simulink model "simulation_block"  (R2024b)
settings: Solver=VariableStepAuto  StartTime=0.0  StopTime=10.0  RelTol=1e-3
undefined symbols (not defined in the file or in its folder): r_min
settings Model: Creator=tianhaoji  LastModifiedBy=tianhaoji

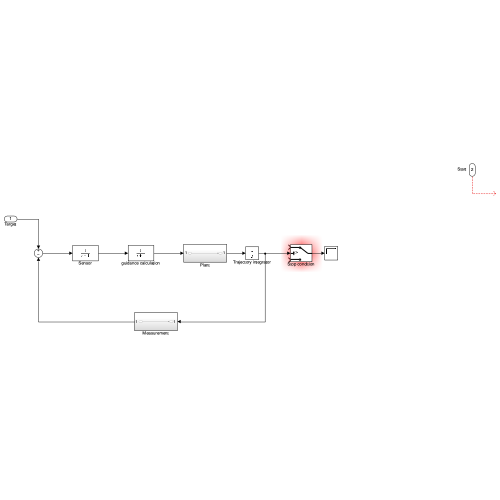
[thumbnail: Simulink's stored preview of the top-level diagram]
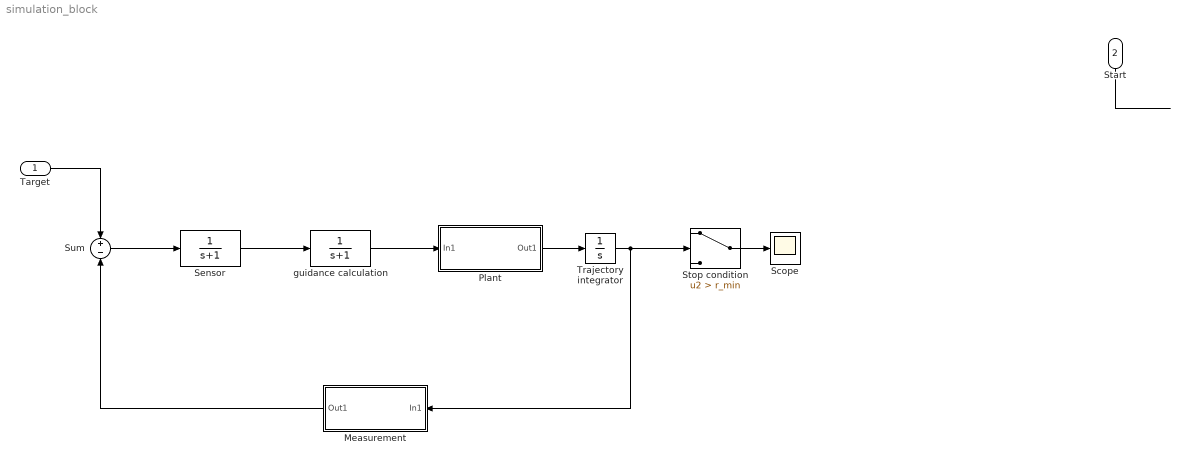
== system simulation_block ==
  Target : Inport
  Start : Inport  Port=2
  Measurement : Subsystem
  Plant : Subsystem
  Scope : Scope
  Sensor : TransferFcn  Denominator=[1 1]
  Stop condition : Switch  Criteria=u2 > Threshold  Threshold=r_min  SaturateOnIntegerOverflow=off  InputSameDT=off
  Sum : Sum  Inputs=+-
  Trajectory integrator : Integrator
  guidance calculation : TransferFcn  Denominator=[1 1]
  wires:
  Target/1 -> Sum/1
  Sum/1 -> Sensor/1
  Sensor/1 -> guidance calculation/1
  guidance calculation/1 -> Plant/1(In1)
  Plant/1(Out1) -> Trajectory integrator/1
  Trajectory integrator/1 -> Stop condition/2, Measurement/1(In1)
  Measurement/1(Out1) -> Sum/2
  Start/1 -> ?
  Stop condition/1 -> Scope/1

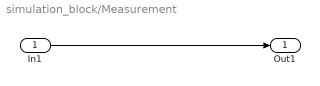
== system simulation_block/Measurement ==
  In1 : Inport
  Out1 : Outport
  wires:
  In1/1 -> Out1/1

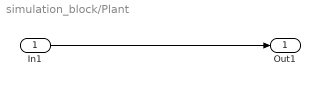
== system simulation_block/Plant ==
  In1 : Inport
  Out1 : Outport
  wires:
  In1/1 -> Out1/1
